simulink model "PolyfitEx"  (R2015a)
settings: Solver=FixedStepDiscrete  StartTime=0.0  StopTime=50  FixedStep=0.2  RelTol=1e-3
values from neighbouring files (symbols this model uses):
  X = [0:0.1:10]    [run_PolyfitEx.m]
  x = [0 1 2   3 5   6 7 8 9 10]    [run_PolyfitEx.m]
  y0 = [1 2 2.5 3 3.5 5 7 6 7 8]    [run_PolyfitEx.m]
libraries: lib_GenTools_PolynomialFit x1
settings Model: Creator=jlkratz  LastModifiedBy=jlkratz

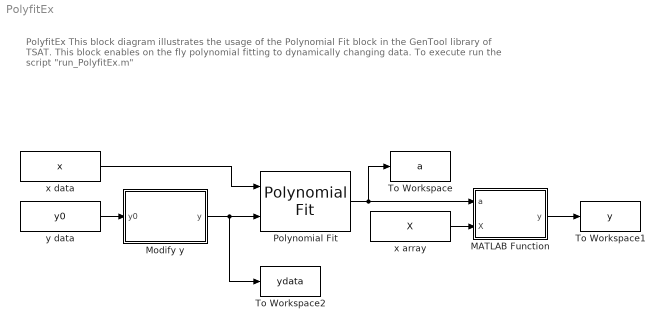
== system PolyfitEx ==
  note: PolyfitEx
      |
      | This block diagram illustrates the usage of the Polynomial Fit block in the GenTool library of TSAT. This
      | block enables on the fly polynomial fitting to dynamically changing data.
      |
      | To execute run the script "run_PolyfitEx.m"
  MATLAB Function : MATLAB Function  TreatAsAtomicUnit=on
  Modify y : Subsystem
  Polynomial Fit : lib_GenTools_PolynomialFit/Polynomial Fit  N_M=6  BN_M=double(gcb)
  To Workspace : ToWorkspace  VariableName=a  SaveFormat=Timeseries  SampleTime=-1
  To Workspace1 : ToWorkspace  VariableName=y  SaveFormat=Timeseries  SampleTime=-1
  To Workspace2 : ToWorkspace  VariableName=ydata  SaveFormat=Timeseries  SampleTime=-1
  x array : Constant  Value=X
  x data : Constant  Value=x
  y data : Constant  Value=y0
  wires:
  y data/1 -> Modify y/1(y0)
  Modify y/1(y) -> To Workspace2/1, Polynomial Fit/2
  x data/1 -> Polynomial Fit/1
  Polynomial Fit/1 -> To Workspace/1, MATLAB Function/1(a)
  x array/1 -> MATLAB Function/2(X)
  MATLAB Function/1(y) -> To Workspace1/1

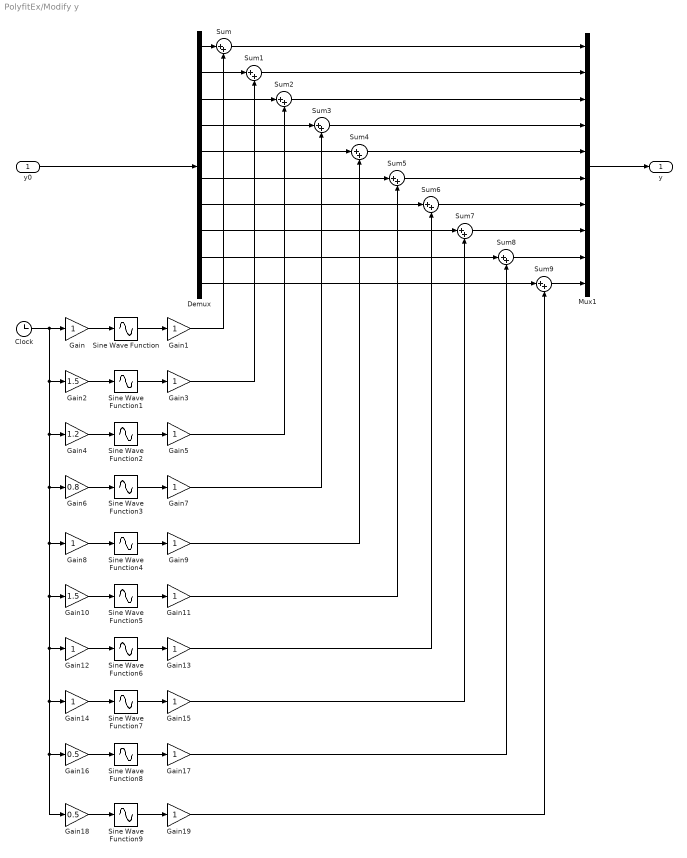
== system PolyfitEx/Modify y ==
  y0 : Inport
  Clock : Clock
  Demux : Demux  Outputs=10
  Gain{,1,3,5,7..9,11..15,17,19} (14 alike) : Gain
  Gain10 : Gain  Gain=1.5
  Gain16 : Gain  Gain=0.5
  Gain18 : Gain  Gain=0.5
  Gain2 : Gain  Gain=1.5
  Gain4 : Gain  Gain=1.2
  Gain6 : Gain  Gain=0.8
  Mux1 : Mux  Inputs=10
  Sine Wave Function{,1..9} (10 alike) : Sin  TimeSource=Use external signal  SampleTime=0
  Sum{,1..9} (10 alike) : Sum  Inputs=|++
  y : Outport
  wires:
  Gain18/1 -> Sine Wave Function9/1
  Sine Wave Function9/1 -> Gain19/1
  Gain10/1 -> Sine Wave Function5/1
  Sine Wave Function5/1 -> Gain11/1
  Gain8/1 -> Sine Wave Function4/1
  Mux1/1 -> y/1
  y0/1 -> Demux/1
  Gain14/1 -> Sine Wave Function7/1
  Sine Wave Function7/1 -> Gain15/1
  Sine Wave Function4/1 -> Gain9/1
  Gain6/1 -> Sine Wave Function3/1
  Sum9/1 -> Mux1/10
  Demux/7 -> Sum6/1
  Clock/1 -> Gain18/1, Gain16/1, Gain14/1, Gain12/1, Gain10/1, Gain8/1, Gain6/1, Gain4/1, Gain2/1, Gain/1
  Gain/1 -> Sine Wave Function/1
  Sine Wave Function6/1 -> Gain13/1
  Gain16/1 -> Sine Wave Function8/1
  Gain12/1 -> Sine Wave Function6/1
  Gain2/1 -> Sine Wave Function1/1
  Demux/10 -> Sum9/1
  Gain4/1 -> Sine Wave Function2/1
  Sine Wave Function1/1 -> Gain3/1
  Sine Wave Function8/1 -> Gain17/1
  Sum5/1 -> Mux1/6
  Demux/4 -> Sum3/1
  Sine Wave Function3/1 -> Gain7/1
  Demux/1 -> Sum/1
  Demux/5 -> Sum4/1
  Demux/6 -> Sum5/1
  Demux/2 -> Sum1/1
  Demux/8 -> Sum7/1
  Demux/3 -> Sum2/1
  Demux/9 -> Sum8/1
  Sine Wave Function2/1 -> Gain5/1
  Sine Wave Function/1 -> Gain1/1
  Gain5/1 -> Sum2/2
  Gain3/1 -> Sum1/2
  Sum4/1 -> Mux1/5
  Gain7/1 -> Sum3/2
  Gain13/1 -> Sum6/2
  Sum/1 -> Mux1/1
  Sum7/1 -> Mux1/8
  Gain17/1 -> Sum8/2
  Sum8/1 -> Mux1/9
  Gain1/1 -> Sum/2
  Sum1/1 -> Mux1/2
  Gain9/1 -> Sum4/2
  Gain11/1 -> Sum5/2
  Gain19/1 -> Sum9/2
  Sum2/1 -> Mux1/3
  Sum6/1 -> Mux1/7
  Sum3/1 -> Mux1/4
  Gain15/1 -> Sum7/2

== matlab function PolyfitEx/MATLAB Function ==
  data: a input; y output; X input
function y = fcn(a,X)
%#codegen

y = a(1) + a(2)*X + a(3)*X.^2 + a(4)*X.^3 + a(5)*X.^4 ...
    + a(6)*X.^5 + a(7)*X.^6;
